simulink model "sim_Ex9"  (R2022b)
settings: Solver=FixedStepAuto  StartTime=0.0  StopTime=inf  FixedStep=1e-3
libraries: simulink x5
settings Model: Creator=MAAM  LastModifiedBy=MAAM
settings OptimizationCC: DefaultParameterBehavior=Inlined  UseDivisionForNetSlopeComputation=on  GainParamInheritBuiltInType=on  UseFloatMulNetSlope=on  InlineInvariantSignals=on  PassReuseOutputArgsAs=Individual arguments  ZeroExternalMemoryAtStartup=off  ZeroInternalMemoryAtStartup=off  NoFixptDivByZeroProtection=on  EfficientFloat2IntCast=on  LifeSpan=1  OptimizeBlockOrder=speed  DifferentSizesBufferReuse=on  EfficientTunableParamExpr=on
settings DebuggingCC: ParameterTunabilityLossMsg=error
settings HardwareCC: ProdLongLongMode=on
settings SFSimCC: MATLABDynamicMemAlloc=off
settings RTWCC: Description=Embedded Coder  SystemTargetFile=ert.tlc  TemplateMakefile=ert_default_tmf
settings CodeAppCC: ForceParamTrailComments=on  IgnoreCustomStorageClasses=off  OperatorAnnotations=on  SimulinkDataObjDesc=on  SFDataObjDesc=on  CustomSymbolStrGlobalVar=rt$N$M  CustomSymbolStrType=$N$M  CustomSymbolStrFcn=$N$M$F  CustomSymbolStrMacro=$N$M  InsertBlockDesc=on
settings ERTTargetCC: TargetLangStandard=C99 (ISO)  GenerateSampleERTMain=on  IncludeMdlTerminateFcn=off  CombineSignalStateStructs=on  SupportComplex=off  SupportContinuousTime=on  InlinedParameterPlacement=NonHierarchical  ERTCustomFileTemplate=example_file_process.tlc  ERTFilePackagingFormat=CompactWithDataFile

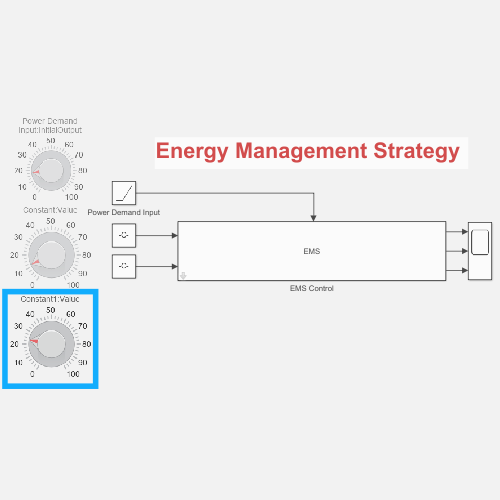
[thumbnail: Simulink's stored preview of the top-level diagram]
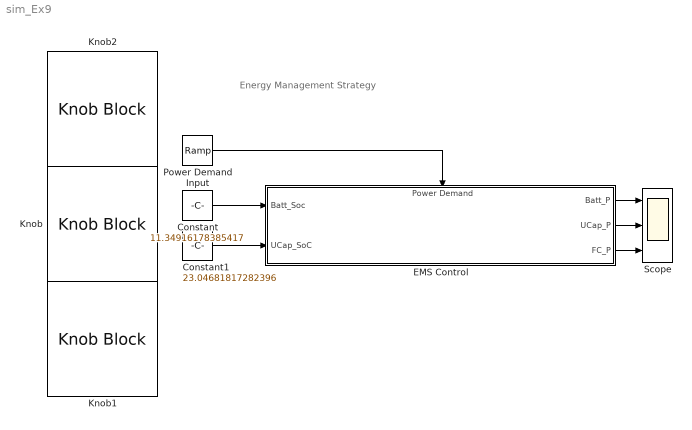
== system sim_Ex9 ==
  note: Energy Management Strategy
  Constant : Constant  Value=11.34916178385417
  Constant1 : Constant  Value=23.04681817282396
  EMS Control : Subsystem  mask{LowerLimmit=33, UpperLimmit=55, Batt_SoC_Min=10, UCap_SoC_Min=10}
      mask prompts: LowerLimmit "Power Demand Lower Limmit (KW)"; UpperLimmit "Power Demand Upper Limmit (KW)"; Batt_SoC_Min "Battary Minimum SoC"; UCap_SoC_Min "Ultracapacitor Minimum SoC"
      settings: PortSchema="{\"entries\":[{\"content\":{\"sides\":[{\"content\":{\"connectorIds\":[\"In1\",\"In2\"]},\"type\":\"ConnectorPlacement.EquallySpacedRectSide\",\"uuid\":\"2460d459-b836-4198-97db-aed0de2a7119\"},{\"content\":{\"connectorIds\":[\"Out1\",\"Out2\",\"Out3\"],\"side\":\"RIGHT\"},\"type\":\"ConnectorPlacement.EquallySpacedRectSide\",\"uuid\":\"9da73925-4d5b-4b1b-8e01-cb3524c7ce04\"},{\"content\":{\"connectorIds\":[\"In3\"],\"side\":\"TOP\"},\"type\":\"ConnectorPlacement.EquallySpacedRectSide\",\"uuid\":\"ed3d53ec-cf4c-41f0-8caf-be13cb737280\"},{\"content\":{\"connectorIds\":[],\"side\":\"BOTTOM\"},\"type\":\"ConnectorPlacement.EquallySpacedRectSide\",\"uuid\":\"a8349bc6-5458-4711-afed-81828516a425\"}]},\"type\":\"ConnectorPlacement.EquallySpacedConnector\",\"uuid\":\"6ea30aae-0445-446b-b280-0d4384085239\"}],\"packageUris\":[\"http://schema.mathworks.com/mf0/Connector/R2020b\"],\"version\":\"1.0\"}"
      mask Display: fprintf('EMS');
  Knob : KnobBlock
  Knob1 : KnobBlock
  Knob2 : KnobBlock
  Power Demand Input : simulink/Sources/Ramp  slope=10  start=0  InitialOutput=17.49534606933594
  Scope : Scope  NumInputPorts=3
  wires:
  Power Demand Input/1 -> EMS Control/3(Power Demand)
  EMS Control/1(Batt_P) -> Scope/1
  EMS Control/2(UCap_P) -> Scope/2
  EMS Control/3(FC_P) -> Scope/3
  Constant/1 -> EMS Control/1(Batt_Soc)
  Constant1/1 -> EMS Control/2(UCap_SoC)

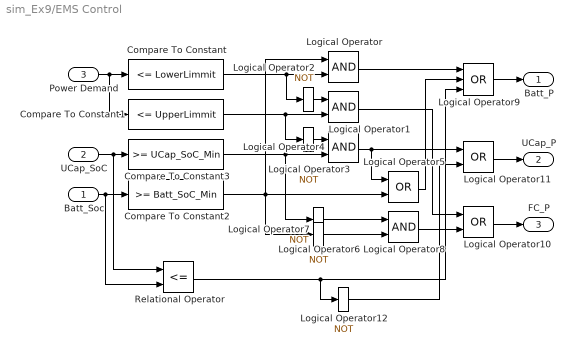
== system sim_Ex9/EMS Control ==
  Batt_Soc : Inport
  UCap_SoC : Inport  Port=2
  Power Demand : Inport  Port=3
  Compare To Constant : simulink/Logic and Bit Operations/Compare To Constant  relop=<=  const=LowerLimmit  OutDataTypeStr=boolean
  Compare To Constant1 : simulink/Logic and Bit Operations/Compare To Constant  relop=<=  const=UpperLimmit  OutDataTypeStr=boolean
  Compare To Constant2 : simulink/Logic and Bit Operations/Compare To Constant  relop=>=  const=Batt_SoC_Min  OutDataTypeStr=boolean
  Compare To Constant3 : simulink/Logic and Bit Operations/Compare To Constant  relop=>=  const=UCap_SoC_Min  OutDataTypeStr=boolean
  Logical Operator{,1,4,8} (4 alike) : Logic  AllPortsSameDT=off  OutDataTypeStr=boolean
  Logical Operator10 : Logic  Operator=OR  AllPortsSameDT=off  OutDataTypeStr=boolean
  Logical Operator11 : Logic  Operator=OR  AllPortsSameDT=off  OutDataTypeStr=boolean
  Logical Operator{2..3,6..7,12} (5 alike) : Logic  Operator=NOT  IconShape=distinctive  AllPortsSameDT=off  OutDataTypeStr=boolean
  Logical Operator5 : Logic  Operator=OR  AllPortsSameDT=off  OutDataTypeStr=boolean
  Logical Operator9 : Logic  Operator=OR  Inputs=3  AllPortsSameDT=off  OutDataTypeStr=boolean
  Relational Operator : RelationalOperator  Operator=<=  OutDataTypeStr=boolean  RndMeth=Simplest  InputSameDT=off
  Batt_P : Outport
  UCap_P : Outport  Port=2
  FC_P : Outport  Port=3
  wires:
  Power Demand/1 -> Compare To Constant1/1, Compare To Constant/1
  Compare To Constant/1 -> Logical Operator2/1, Logical Operator/2
  Compare To Constant1/1 -> Logical Operator3/1, Logical Operator1/2
  Batt_Soc/1 -> Relational Operator/2, Compare To Constant2/1
  Compare To Constant2/1 -> Logical Operator5/2, Logical Operator7/1, Logical Operator/1
  Logical Operator2/1 -> Logical Operator1/1
  Logical Operator3/1 -> Logical Operator4/1
  UCap_SoC/1 -> Relational Operator/1, Compare To Constant3/1
  Compare To Constant3/1 -> Logical Operator6/1, Logical Operator4/2
  Logical Operator4/1 -> Logical Operator5/1, Logical Operator11/1
  Logical Operator6/1 -> Logical Operator8/1
  Logical Operator7/1 -> Logical Operator8/2
  Logical Operator/1 -> Logical Operator9/1
  Logical Operator5/1 -> Logical Operator9/2
  Logical Operator8/1 -> Logical Operator10/2
  Logical Operator1/1 -> Logical Operator10/1
  Logical Operator9/1 -> Batt_P/1
  Logical Operator10/1 -> FC_P/1
  Relational Operator/1 -> Logical Operator12/1, Logical Operator9/3
  Logical Operator11/1 -> UCap_P/1
  Logical Operator12/1 -> Logical Operator11/2
